simulink model "WiperSystem"  (R2022a)
settings: Solver=FixedStepDiscrete  StartTime=0.0  StopTime=20  FixedStep=0.01  RelTol=1e-3
model workspace (MAT data in the model file):
  x_data = Simulink.Parameter
  x_data.Value = [0; 1; 2; 3; 4; 5; 6; 7]
  x_data.DataType = 'uint8'
  x_data.Complexity = 'real'
  x_data.Dimensions = [8 1]
  y_data = Simulink.Parameter
  y_data.Value = [0; 0.4; 0.45; 0.5; 0.55; 0.6; 0.65; 0.7]
  y_data.DataType = 'single'
  y_data.Complexity = 'real'
  y_data.Dimensions = [8 1]
undefined symbols (not defined in the file): sigbuilder_block
libraries: simulink x1
settings Model: Creator=amiru  LastModifiedBy=amiru

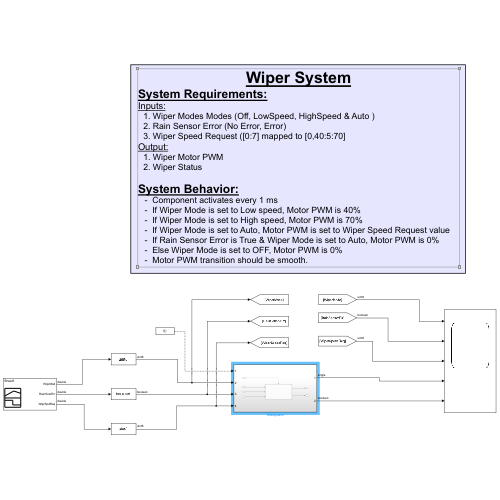
[thumbnail: Simulink's stored preview of the top-level diagram]
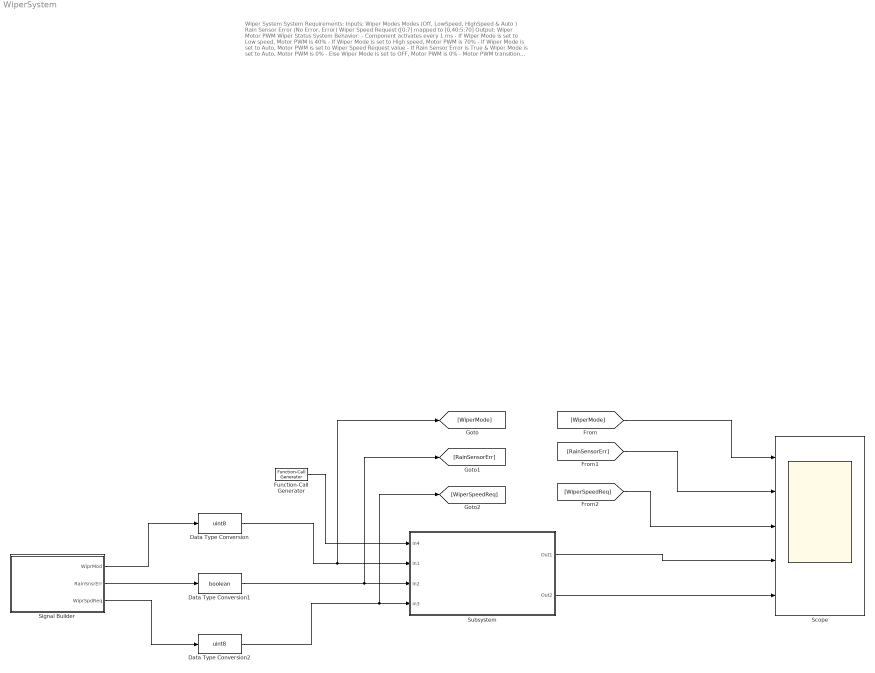
== system WiperSystem ==
  note: Wiper System
      | System Requirements:
      | Inputs:
      | Wiper Modes Modes (Off, LowSpeed, HighSpeed & Auto )
      | Rain Sensor Error (No Error, Error)
      | Wiper Speed Request ([0:7] mapped to [0,40:5:70]
      | Output:
      | Wiper Motor PWM
      | Wiper Status
      |
      | System Behavior:
      | - Component activates every 1 ms
      | - If Wiper Mode is set to Low speed, Motor PWM is 40%
      | - If Wiper Mode is set to High speed, Motor PWM is 70%
      | - If Wiper Mode is set to Auto, Motor PWM is set to Wiper Speed Request value
      | - If Rain Sensor Error is True & Wiper Mode is set to Auto, Motor PWM is 0%
      | - Else Wiper Mode is set to OFF, Motor PWM is 0%
      | - Motor PWM transition should be smooth.
  Data Type Conversion : DataTypeConversion  OutMin=0  OutMax=3  OutDataTypeStr=uint8  SaturateOnIntegerOverflow=off  RndMeth=Floor
  Data Type Conversion1 : DataTypeConversion  OutMin=0  OutMax=1  OutDataTypeStr=boolean  SaturateOnIntegerOverflow=off  RndMeth=Floor
  Data Type Conversion2 : DataTypeConversion  OutMin=0  OutMax=7  OutDataTypeStr=uint8  SaturateOnIntegerOverflow=off  RndMeth=Floor
  Function-Call Generator : simulink/Ports & Subsystems/Function-Call Generator  sample_time=10e-3  numberOfIterations=1  DisallowWideOutput=off
  Scope : Scope  NumInputPorts=5
  Signal Builder : Subsystem  Tag=STV Subsys  LoadFcn=sigbuilder_block('load');  StartFcn=sigbuilder_block('start');  StopFcn=sigbuilder_block('stop');  ClipboardFcn=sigbuilder_block('clipboard');  mask(Sigbuilder block){tuvar=[0:10]}
      mask help: Simulink:masks:SigbuilderBlock_MD
      mask init:
      | if ~strcmp(get_param(bdroot(gcbh),'SimulationStatus'),'stopped') tuvar = sigbuilder_block('maskInit'); end
      settings: CopyFcn=sigbuilder_block('copy');  DeleteFcn=sigbuilder_block('delete');  ModelCloseFcn=sigbuilder_block('modelClose');  PreSaveFcn=sigbuilder_block('preSave');  PauseFcn=sigbuilder_block('pause');  ContinueFcn=sigbuilder_block('continue');  NameChangeFcn=sigbuilder_block('namechange');  OpenFcn=sigbuilder_block('open',[428.4 165 601.8 400.2 ]);  CloseFcn=sigbuilder_block('close');
      mask Display: plot(0, 0, 100, 100,[2, 2, 32, 32, 2], [68, 8, 8, 68, 68],[32, 2], [38, 38], [32, 19, 2],[53, 60, 44], [32, 17, 17, 2],[16, 16, 31, 31]);txt = getActiveGroup(gcbh);text(2, 100, txt,'verticalAlignment', 'top');
  Subsystem : Subsystem
  wires:
  Function-Call Generator/1 -> Subsystem/1(In4)
  Signal Builder/1(WiprMod) -> Data Type Conversion/1
  Signal Builder/2(RainSnsrErr) -> Data Type Conversion1/1
  Signal Builder/3(WiprSpdReq) -> Data Type Conversion2/1
  Data Type Conversion/1 -> [WiperMode], Subsystem/2(In1)
  Data Type Conversion1/1 -> [RainSensorErr], Subsystem/3(In2)
  Data Type Conversion2/1 -> [WiperSpeedReq], Subsystem/4(In3)
  [WiperMode] -> Scope/1
  [RainSensorErr] -> Scope/2
  [WiperSpeedReq] -> Scope/3
  Subsystem/1(Out1) -> Scope/4
  Subsystem/2(Out2) -> Scope/5

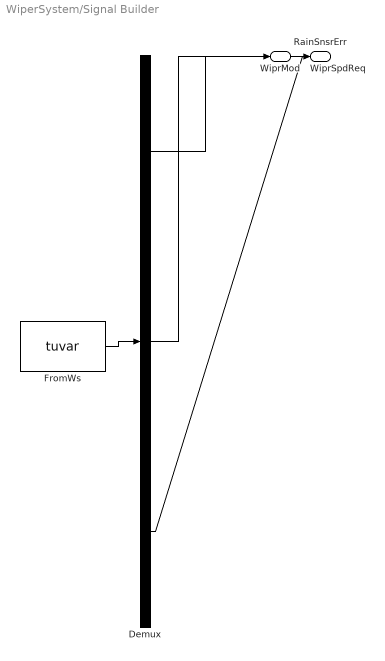
== system WiperSystem/Signal Builder ==
  Demux : Demux  Tag=STV Demux  Outputs=3
      settings: DisplayOption=none
  FromWs : FromWorkspace  Tag=STV FromWs  VariableName=tuvar
      SigBuilderData=|
      | common.afterFinalStr = 'Extrapolate'
      | common.sampleTime = 0
      | dataSet.timeRange = [0 20]
      | dataSet.name = 'Sheet1'
      | sbobj.Name = 'Signal Builder'
      | sbobj.Groups.Name = 'Sheet1'
      | sbobj.Groups.Signals(1).Name = 'WiprMod'
      | sbobj.Groups.Signals(1).XData = [0 1 2 3 4 5 6 7 8 9 10 11 12 13 14 15 20]
      | sbobj.Groups.Signals(1).YData = [0 0 2 2 3 3 1 1 1 1 1 1 1 1 1 1 1]
      | sbobj.Groups.Signals(2).Name = 'RainSnsrErr'
      | sbobj.Groups.Signals(2).XData = [0 1 2 3 4 5 6 7 8 9 10 11 12 13 14 15 16 20]
      | sbobj.Groups.Signals(2).YData = [0 0 0 0 0 0 0 0 0 0 0 0 0 0 0 1 0 0]
      | sbobj.Groups.Signals(3).Name = 'WiprSpdReq'
      | sbobj.Groups.Signals(3).XData = [0 1 2 3 4 5 6 7 8 9 10 11 12 13 14 15 20]
      | sbobj.Groups.Signals(3).YData = [0 0 0 0 0 0 0 0 1 2 3 4 5 6 7 7 7]
      | sbobj.Groups.TimeRange = [0 20]
  WiprMod : Outport  Tag=STV Outport
  RainSnsrErr : Outport  Tag=STV Outport  Port=2
  WiprSpdReq : Outport  Tag=STV Outport  Port=3
  wires:
  Demux/1 -> WiprMod/1
  FromWs/1 -> Demux/1
  Demux/2 -> RainSnsrErr/1
  Demux/3 -> WiprSpdReq/1

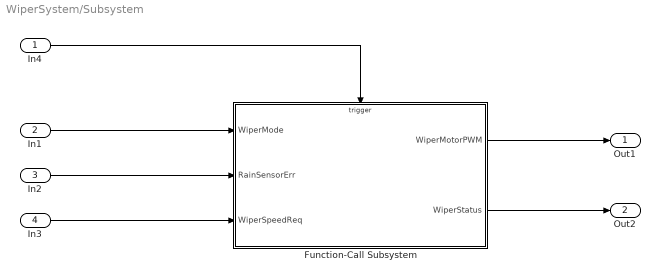
== system WiperSystem/Subsystem ==
  In4 : Inport
  In1 : Inport  Port=2  OutMin=0  OutMax=3
  In2 : Inport  Port=3  OutMin=0  OutMax=1
  In3 : Inport  Port=4  OutMin=0  OutMax=7
  Function-Call Subsystem : Subsystem  TreatAsAtomicUnit=on
  Out1 : Outport  OutMin=0  OutMax=1  OutDataTypeStr=single
  Out2 : Outport  Port=2  OutMin=0  OutMax=1  OutDataTypeStr=boolean
  wires:
  In1/1 -> Function-Call Subsystem/1(WiperMode)
  Function-Call Subsystem/2(WiperStatus) -> Out2/1
  In4/1 -> Function-Call Subsystem/Trigger
  In2/1 -> Function-Call Subsystem/2(RainSensorErr)
  In3/1 -> Function-Call Subsystem/3(WiperSpeedReq)
  Function-Call Subsystem/1(WiperMotorPWM) -> Out1/1

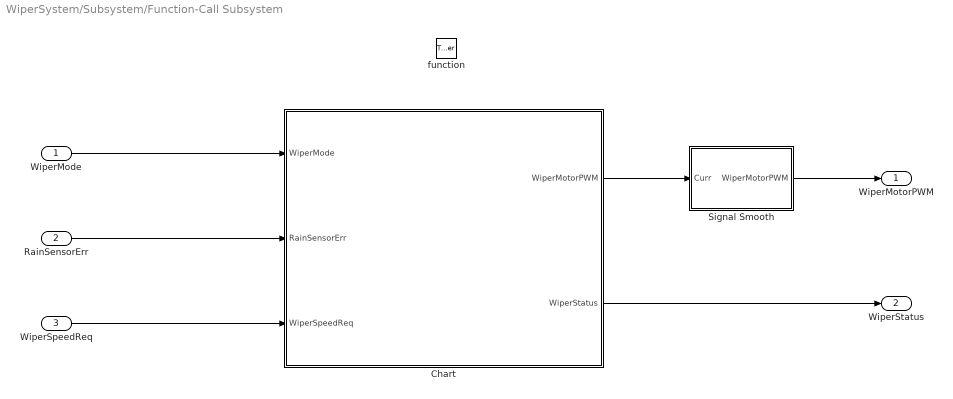
== system WiperSystem/Subsystem/Function-Call Subsystem ==
  WiperMode : Inport  OutMin=0  OutMax=3  OutDataTypeStr=uint8
  RainSensorErr : Inport  Port=2  OutMin=0  OutMax=1  OutDataTypeStr=boolean
  WiperSpeedReq : Inport  Port=3  OutMin=0  OutMax=7  OutDataTypeStr=uint8
  function : TriggerPort  TriggerType=function-call  VariantControl=(inherit)
  Chart : Stateflow chart  TreatAsAtomicUnit=on
  Signal Smooth : Subsystem
  WiperMotorPWM : Outport  OutMin=0  OutMax=1  OutDataTypeStr=single
  WiperStatus : Outport  Port=2  OutMin=0  OutMax=1  OutDataTypeStr=boolean
  wires:
  WiperMode/1 -> Chart/1(WiperMode)
  RainSensorErr/1 -> Chart/2(RainSensorErr)
  WiperSpeedReq/1 -> Chart/3(WiperSpeedReq)
  Chart/2(WiperStatus) -> WiperStatus/1
  Chart/1(WiperMotorPWM) -> Signal Smooth/1(Curr)
  Signal Smooth/1(WiperMotorPWM) -> WiperMotorPWM/1

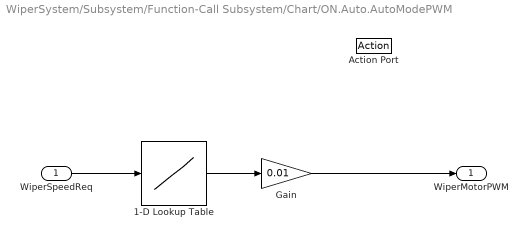
== system WiperSystem/Subsystem/Function-Call Subsystem/Chart/ON.Auto.AutoModePWM ==
  WiperSpeedReq : Inport  OutDataTypeStr=uint8
  Action Port : ActionPort
      settings: CopyFcn=Stateflow.SLINSF.SimulinkMan.removeBlockPreDeleteFcn  PreDeleteFcn=Stateflow.SLINSF.SimulinkMan.unsafePredeleteFcn
  1-D Lookup Table : Lookup_n-D  NumberOfTableDimensions=1  BreakpointsForDimension1=[0;1;2;3;4;5;6;7]  Table=[0;40;45;50;55;60;65;70]  TableDataTypeStr=single  ExtrapMethod=Clip  InternalRulePriority=Speed  OutDataTypeStr=single  RndMeth=Simplest
  Gain : Gain  Gain=0.01  OutDataTypeStr=Inherit: Inherit via back propagation
  WiperMotorPWM : Outport
  wires:
  WiperSpeedReq/1 -> 1-D Lookup Table/1
  1-D Lookup Table/1 -> Gain/1
  Gain/1 -> WiperMotorPWM/1

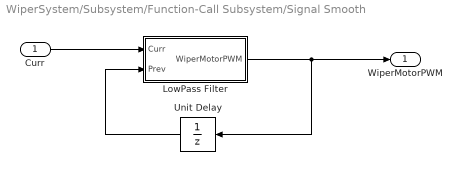
== system WiperSystem/Subsystem/Function-Call Subsystem/Signal Smooth ==
  Curr : Inport
  LowPass Filter : Subsystem
  Unit Delay : UnitDelay  SampleTime=-1  HasFrameUpgradeWarning=on
  WiperMotorPWM : Outport
  wires:
  LowPass Filter/1(WiperMotorPWM) -> WiperMotorPWM/1, Unit Delay/1
  Unit Delay/1 -> LowPass Filter/2(Prev)
  Curr/1 -> LowPass Filter/1(Curr)

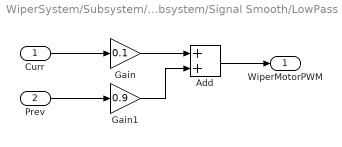
== system WiperSystem/Subsystem/Function-Call Subsystem/Signal Smooth/LowPass Filter ==
  Curr : Inport
  Prev : Inport  Port=2
  Add : Sum
  Gain : Gain  Gain=0.1
  Gain1 : Gain  Gain=0.9
  WiperMotorPWM : Outport
  wires:
  Curr/1 -> Gain/1
  Gain/1 -> Add/1
  Prev/1 -> Gain1/1
  Gain1/1 -> Add/2
  Add/1 -> WiperMotorPWM/1

== stateflow chart WiperSystem/Subsystem/Function-Call Subsystem/Chart ==
  state ON
    state Auto
      during:
      WiperStatus = true;
      state AutoModePWM
      (default) -> AutoModePWM
    state LoSpeed
      entry:
      WiperStatus = true;
      WiperMotorPWM = 0.4;
    state HiSpeed
      entry:
      WiperStatus = true;
      WiperMotorPWM = 0.7;
    (default) -> Auto [commented out]
    (junction 43) -> Auto [order 1]
    LoSpeed -> Auto [order 1] : [WiperMode == 1]
    Auto -> LoSpeed [order 1] : [WiperMode == 2]
    Auto -> HiSpeed [order 3] : [WiperMode == 3]
    HiSpeed -> Auto [order 2] : [WiperMode==1]
    LoSpeed -> HiSpeed [order 2] : [WiperMode == 3]
    (junction 43) -> HiSpeed [order 3] : [WiperMode == 3]
    (default) -> (junction 43)
    (junction 43) -> LoSpeed [order 2] : [WiperMode == 2]
    HiSpeed -> LoSpeed [order 1] : [WiperMode == 2]
  state OFF
    entry:
    WiperMotorPWM = 0;
    WiperStatus = false;
  (default) -> OFF
  OFF -> ON : [WiperMode~=0 && RainSensorErr==0]
  ON -> OFF : [WiperMode==0]
  Auto -> OFF [order 2] : [WiperMotorPWM == 0 ||RainSensorErr == 1]
  data: sf_internal_action_state_placeholder_data local double size=1 =0; WiperMode input; RainSensorErr input; WiperSpeedReq input; WiperMotorPWM output single; WiperStatus output boolean
